simulink model "LunarLanderLQRAndObserverIntegralAction"  (R2022b)
settings: Solver=ode45  StartTime=0.0  StopTime=35  RelTol=1e-2
undefined symbols (not defined in the file): A, B, C, Kp, L
settings Model: Creator=marco  LastModifiedBy=marco

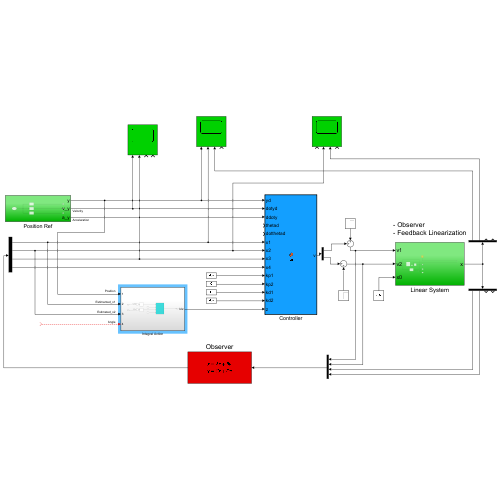
[thumbnail: Simulink's stored preview of the top-level diagram]
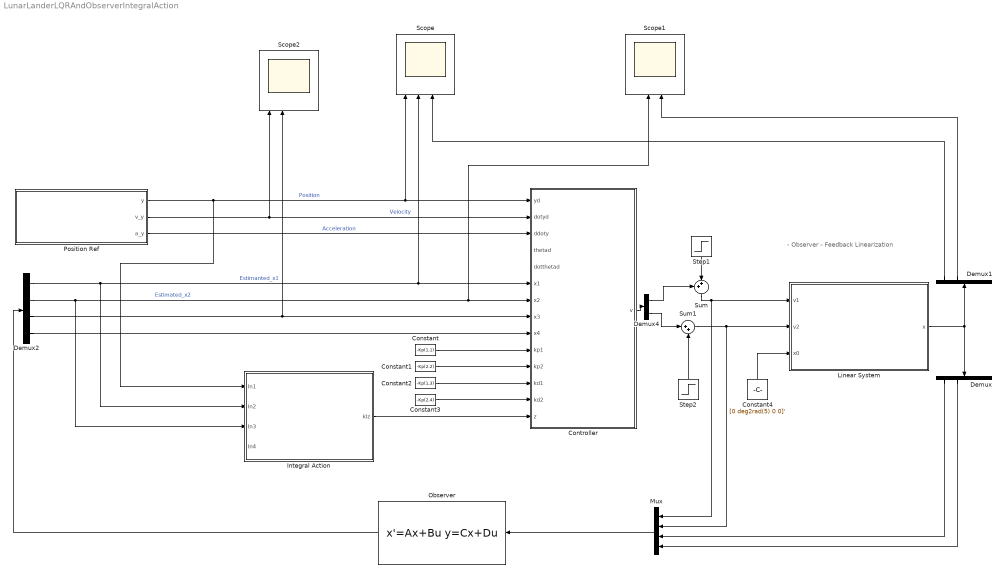
== system LunarLanderLQRAndObserverIntegralAction ==
  note: - Observer
      | - Feedback Linearization
  Constant : Constant  Value=-Kp(1,1)
  Constant1 : Constant  Value=-Kp(2,2)
  Constant2 : Constant  Value=-Kp(1,3)
  Constant3 : Constant  Value=-Kp(2,4)
  Constant4 : Constant  Value=[0 deg2rad(5) 0 0]'
  Controller : MATLAB Function  TreatAsAtomicUnit=on
  Demux : Demux
  Demux1 : Demux
  Demux2 : Demux
  Demux4 : Demux  Outputs=2
  Integral Action : Subsystem
  Linear System : Subsystem
  Mux : Mux
  Observer : StateSpace  A=A-L*C  B=[B L]  C=eye(4)  D=zeros(4)  InitialCondition=0
  Position Ref : Subsystem
  Scope : Scope  NumInputPorts=4
  Scope1 : Scope  NumInputPorts=4
  Scope2 : Scope  NumInputPorts=4
  Step1 : Step  After=10  SampleTime=0
  Step2 : Step  After=deg2rad(1)  SampleTime=0
  Sum : Sum  Inputs=++|
  Sum1 : Sum  Inputs=|++
  wires:
  Demux2/4 -> Controller/9(x4)
  Demux/1 -> Mux/3
  Sum/1 -> Mux/1, Linear System/1(v1)
  Linear System/1(x) -> Demux/1, Demux1/1
  Step2/1 -> Sum1/2
  Demux2/2 -> Scope1/2, Controller/7(x2), Integral Action/3(In3)  "Estimated_x2"
  Demux2/1 -> Scope/2, Controller/6(x1), Integral Action/2(In2)  "Estimanted_x1"
  Demux1/1 -> Scope/3
  Step1/1 -> Sum/2
  Position Ref/3(a_y) -> Controller/3(ddoty)  "Acceleration"
  Demux2/3 -> Scope2/2, Controller/8(x3)
  Constant2/1 -> Controller/12(kd1)
  Controller/1(v) -> Demux4/1
  Position Ref/2(v_y) -> Scope2/1, Controller/2(dotyd)  "Velocity"
  Integral Action/1(kIz) -> Controller/14(z)
  Constant4/1 -> Linear System/3(x0)
  Demux/2 -> Mux/4
  Constant1/1 -> Controller/11(kp2)
  Sum1/1 -> Mux/2, Linear System/2(v2)
  Demux4/1 -> Sum/1
  Demux4/2 -> Sum1/1
  Constant/1 -> Controller/10(kp1)
  Position Ref/1(y) -> Controller/1(yd), Scope/1, Integral Action/1(In1)  "Position"
  Observer/1 -> Demux2/1
  Constant3/1 -> Controller/13(kd2)
  Mux/1 -> Observer/1
  Demux1/2 -> Scope1/3
  ? -> Integral Action/4(In4)  "Angle"

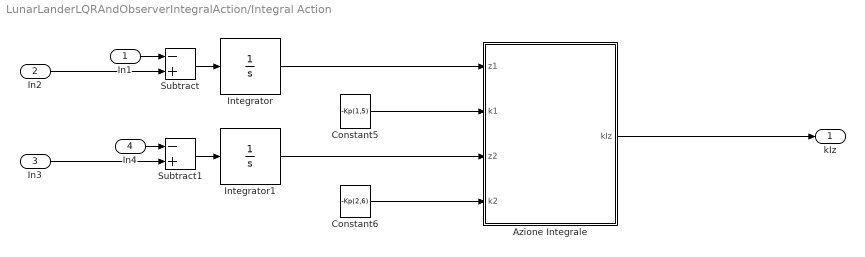
== system LunarLanderLQRAndObserverIntegralAction/Integral Action ==
  In1 : Inport
  In2 : Inport  Port=2
  In3 : Inport  Port=3
  In4 : Inport  Port=4
  Azione Integrale : MATLAB Function  TreatAsAtomicUnit=on
  Constant5 : Constant  Value=-Kp(1,5)
  Constant6 : Constant  Value=-Kp(2,6)
  Integrator : Integrator
  Integrator1 : Integrator
  Subtract : Sum  Inputs=-+
  Subtract1 : Sum  Inputs=-+
  kIz : Outport
  wires:
  Integrator/1 -> Azione Integrale/1(z1)
  Constant6/1 -> Azione Integrale/4(k2)
  Integrator1/1 -> Azione Integrale/3(z2)
  Subtract1/1 -> Integrator1/1
  Constant5/1 -> Azione Integrale/2(k1)
  Subtract/1 -> Integrator/1
  In3/1 -> Subtract1/2
  In4/1 -> Subtract1/1
  In1/1 -> Subtract/1
  Azione Integrale/1(kIz) -> kIz/1
  In2/1 -> Subtract/2

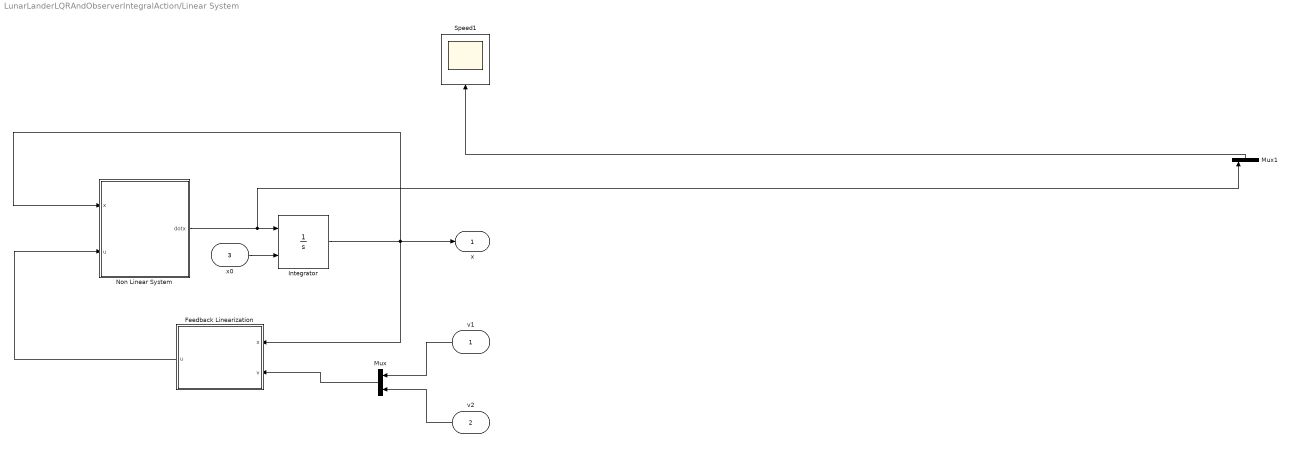
== system LunarLanderLQRAndObserverIntegralAction/Linear System ==
  v1 : Inport
  v2 : Inport  Port=2
  x0 : Inport  Port=3
  Feedback Linearization : MATLAB Function  TreatAsAtomicUnit=on
  Integrator : Integrator  InitialConditionSource=external  InitialCondition=[0 0 0 0]'
  Mux : Mux  Inputs=2
  Mux1 : Mux  Inputs=2
  Non Linear System : MATLAB Function  TreatAsAtomicUnit=on
  Speed1 : Scope
  x : Outport
  wires:
  Feedback Linearization/1(u) -> Non Linear System/2(u)
  Integrator/1 -> Non Linear System/1(x), x/1, Feedback Linearization/1(x)
  Non Linear System/1(dotx) -> Mux1/1, Integrator/1
  x0/1 -> Integrator/2
  v1/1 -> Mux/1
  v2/1 -> Mux/2
  Mux/1 -> Feedback Linearization/2(v)
  Mux1/1 -> Speed1/1

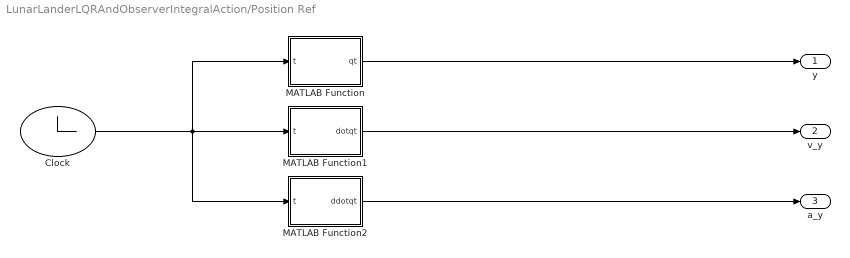
== system LunarLanderLQRAndObserverIntegralAction/Position Ref ==
  Clock : Clock
  MATLAB Function : MATLAB Function  TreatAsAtomicUnit=on
  MATLAB Function1 : MATLAB Function  TreatAsAtomicUnit=on
  MATLAB Function2 : MATLAB Function  TreatAsAtomicUnit=on
  y : Outport
  v_y : Outport  Port=2
  a_y : Outport  Port=3
  wires:
  MATLAB Function/1(qt) -> y/1
  MATLAB Function1/1(dotqt) -> v_y/1
  MATLAB Function2/1(ddotqt) -> a_y/1
  Clock/1 -> MATLAB Function2/1(t), MATLAB Function1/1(t), MATLAB Function/1(t)

== matlab function LunarLanderLQRAndObserverIntegralAction/Linear System/Feedback Linearization ==
  data: x input; v input; u output
function u = fcn(x, v)

g = 1.62;
m = 23000;
J = 100000;
c = 1000;

Q = [sin(x(2))/m cos(x(2))/m;4/J 0]
Qinv = Q^-1

A = [-(g-c*x(3)/m); 0]
ueq = Qinv*(-A+v)

u = [ueq(1); ueq(2)];

== matlab function LunarLanderLQRAndObserverIntegralAction/Linear System/Non Linear System ==
  data: x input; u input; dotx output
function dotx  = fcn(x, u)

g = 1.62;
m = 23000;
J = 100000;
c = 1000;

y = x(1)
theta = x(2)
v = x(3)
w = x(4)

doty = v
dottheta = w
dotv = (u(1)*sin(theta)+u(2)*cos(theta)-m*g-c*v)/m
dotw = 4*u(1)/J

dotx = [doty, dottheta, dotv, dotw]';

== matlab function LunarLanderLQRAndObserverIntegralAction/Controller ==
  data: yd input; dotyd input; ddoty input; thetad input; dotthetad input; x1 input; x2 input; x3 input; x4 input; v output; kp1 input; kp2 input; kd1 input; kd2 input; z input
function v = fcn(yd, dotyd, ddoty, thetad, dotthetad, x1, x2, x3, x4, kp1, kp2, kd1, kd2, z)

v1 = kp1*(x1-yd) + kd1*(x3-dotyd) + ddoty + z(1)
v2 = kp2*(x2-thetad) + kd2*(x4-dotthetad) + z(2)

v = [v1; v2]

== matlab function LunarLanderLQRAndObserverIntegralAction/Integral Action/Azione Integrale ==
  data: z1 input; kIz output; k1 input; z2 input; k2 input
function kIz = fcn(z1, k1, z2, k2)

kIz = [z1*k1; z2*k2];

== matlab function LunarLanderLQRAndObserverIntegralAction/Position Ref/MATLAB Function ==
  data: t input; qt output
function qt = fcn(t)

tf = 20 %s
dotqc = 8 %m/s
qi = 0 %m - valore integratore per y_0
qf = 100 %m

tc = tf - (qf - qi)/dotqc

ddotqc = dotqc/tc

q1 = qi + 0.5 * ddotqc * t^2;
q2 = qi + ddotqc*tc*(t-tc/2);
q3 = qi + ddotqc*tc*(tf-tc-tc/2) + dotqc*(t-(tf-tc))-0.5*ddotqc*(t-(tf-tc))^2;

if t>=0 && t<=tc
    qt = q1
elseif t>tc && t<=(tf-tc)
    qt = q2
elseif t>(tf-tc) && t<=tf
    qt = q3
elseif t>tf
    qt = 100
else 
    qt = 0
end

== matlab function LunarLanderLQRAndObserverIntegralAction/Position Ref/MATLAB Function1 ==
  data: t input; dotqt output
function dotqt = fcn(t)

tf = 20 %s
dotqc = 8 %m/s
qi = 0 %m - valore integratore per y_0
qf = 100 %m

tc = tf - (qf - qi)/dotqc

ddotqc = dotqc/tc

dotq1 = ddotqc*t;
dotq2 = dotqc;
dotq3 = dotqc-ddotqc*(t-(tf-tc));

if t>=0 && t<=tc
    dotqt = dotq1
elseif t>tc && t<=(tf-tc)
    dotqt = dotq2
elseif t>(tf-tc) && t<=tf
    dotqt = dotq3
else 
    dotqt = 0
end

== matlab function LunarLanderLQRAndObserverIntegralAction/Position Ref/MATLAB Function2 ==
  data: t input; ddotqt output
function ddotqt = fcn(t)

tf = 20 %s
dotqc = 8 %m/s
qi = 0 %m - valore integratore per y_0
qf = 100 %m

tc = tf - (qf - qi)/dotqc

ddotqc = dotqc/tc

ddotq1 = ddotqc;
ddotq2 = 0;
ddotq3 = -ddotqc;

if t>=0 && t<=tc
    ddotqt = ddotq1
elseif t>tc && t<=(tf-tc)
    ddotqt = ddotq2
elseif t>(tf-tc) && t<=tf
    ddotqt = ddotq3
else 
    ddotqt = 0
end
